simulink model "simulink_s1_22b"  (R2023b)
settings: Solver=VariableStepAuto  StartTime=0.0  StopTime=45  MaxStep=0.01  RelTol=1e-3
values from neighbouring files (symbols this model uses):
  OUT = [time', Data(:,2)]    [squelette_code_acqui.m]
undefined symbols (not defined in the file or in its folder): REF
settings Model: Creator=Admin  LastModifiedBy=lucasp
settings SolverCC: AlgebraicLoopSolver=TrustRegion

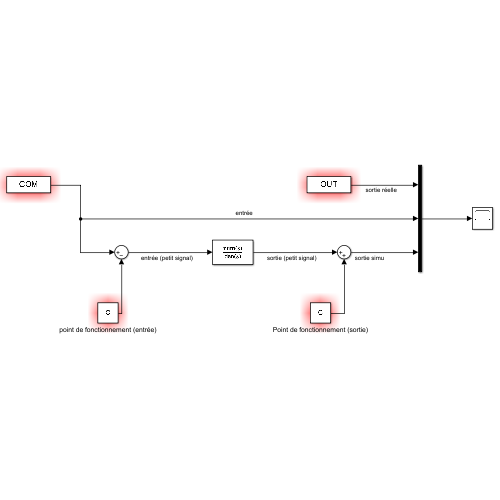
[thumbnail: Simulink's stored preview of the top-level diagram]
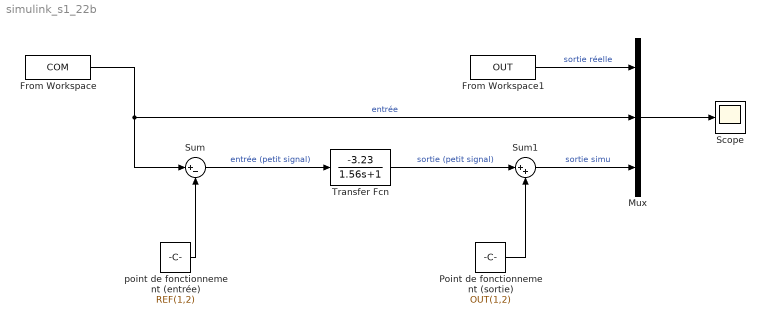
== system simulink_s1_22b ==
  From Workspace : FromWorkspace  VariableName=COM
  From Workspace1 : FromWorkspace  VariableName=OUT
  Mux : Mux  Inputs=3
  Point de fonctionnement (sortie) : Constant  Value=OUT(1,2)
  Scope : Scope
  Sum : Sum  Inputs=|+-
  Sum1 : Sum  Inputs=|++
  Transfer Fcn : TransferFcn  Numerator=[-3.23]  Denominator=[1.56 1]
  point de fonctionnement (entrée) : Constant  Value=REF(1,2)
  wires:
  Sum/1 -> Transfer Fcn/1  "entrée (petit signal)"
  From Workspace1/1 -> Mux/1  "sortie réelle"
  From Workspace/1 -> Sum/1, Mux/2  "entrée"
  Transfer Fcn/1 -> Sum1/1  "sortie (petit signal)"
  Mux/1 -> Scope/1
  Point de fonctionnement (sortie)/1 -> Sum1/2
  point de fonctionnement (entrée)/1 -> Sum/2
  Sum1/1 -> Mux/3  "sortie simu"
